simulink model "GT_trim"  (R2024a)
settings: Solver=ode4  StartTime=0.0  StopTime=t(end)  FixedStep=1/1600  RelTol=1e-3
undefined symbols (not defined in the file): wind_x, wind_y, wind_z
libraries: Sensors x4, GT x1
settings Model: Creator=igmso  LastModifiedBy=igmso
settings DataIOCC: ExternalInput=[t,u]  InitialState=getstatestruct(op_trim3)  LoadExternalInput=on  SaveFormat=StructureWithTime

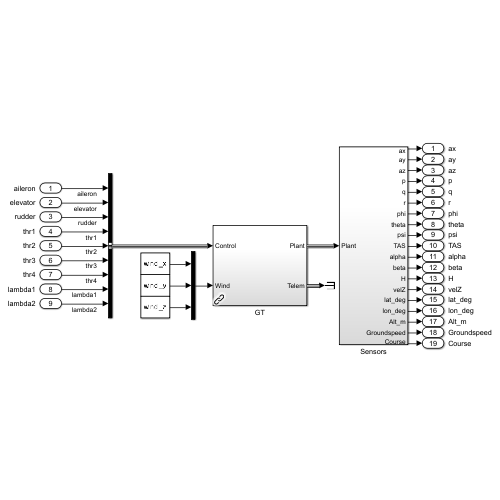
[thumbnail: Simulink's stored preview of the top-level diagram]
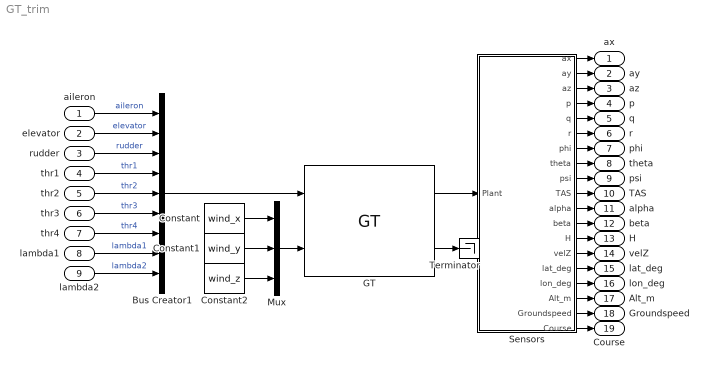
== system GT_trim ==
  aileron : Inport
  elevator : Inport  Port=2
  rudder : Inport  Port=3
  thr1 : Inport  Port=4
  thr2 : Inport  Port=5
  thr3 : Inport  Port=6
  thr4 : Inport  Port=7
  lambda1 : Inport  Port=8
  lambda2 : Inport  Port=9
  Bus Creator1 : BusCreator  Inputs=9
  Constant : Constant  Value=wind_x
  Constant1 : Constant  Value=wind_y
  Constant2 : Constant  Value=wind_z
  GT : GT/GT  SystemSampleTime=-1  VariantActivationTime=update diagram  AllowFlexibleInterface=on  Latency=0  AutoFrameSizeCalculation=off
  Mux : Mux  Inputs=3
  Sensors : Subsystem
  Terminator : Terminator
  ax : Outport
  ay : Outport  Port=2
  az : Outport  Port=3
  p : Outport  Port=4
  q : Outport  Port=5
  r : Outport  Port=6
  phi : Outport  Port=7
  theta : Outport  Port=8
  psi : Outport  Port=9
  TAS : Outport  Port=10
  alpha : Outport  Port=11
  beta : Outport  Port=12
  H : Outport  Port=13
  velZ : Outport  Port=14
  lat_deg : Outport  Port=15
  lon_deg : Outport  Port=16
  Alt_m : Outport  Port=17
  Groundspeed : Outport  Port=18
  Course : Outport  Port=19
  wires:
  Bus Creator1/1 -> GT/1
  lambda2/1 -> Bus Creator1/9  "lambda2"
  lambda1/1 -> Bus Creator1/8  "lambda1"
  thr2/1 -> Bus Creator1/5  "thr2"
  thr3/1 -> Bus Creator1/6  "thr3"
  rudder/1 -> Bus Creator1/3  "rudder"
  thr1/1 -> Bus Creator1/4  "thr1"
  elevator/1 -> Bus Creator1/2  "elevator"
  aileron/1 -> Bus Creator1/1  "aileron"
  thr4/1 -> Bus Creator1/7  "thr4"
  Mux/1 -> GT/2
  Constant/1 -> Mux/1
  Constant1/1 -> Mux/2
  Constant2/1 -> Mux/3
  GT/2 -> Terminator/1
  Sensors/8(theta) -> theta/1
  Sensors/13(H) -> H/1
  Sensors/7(phi) -> phi/1
  Sensors/3(az) -> az/1
  GT/1 -> Sensors/1(Plant)
  Sensors/9(psi) -> psi/1
  Sensors/1(ax) -> ax/1
  Sensors/2(ay) -> ay/1
  Sensors/11(alpha) -> alpha/1
  Sensors/6(r) -> r/1
  Sensors/5(q) -> q/1
  Sensors/4(p) -> p/1
  Sensors/12(beta) -> beta/1
  Sensors/10(TAS) -> TAS/1
  Sensors/16(lon_deg) -> lon_deg/1
  Sensors/14(velZ) -> velZ/1
  Sensors/15(lat_deg) -> lat_deg/1
  Sensors/17(Alt_m) -> Alt_m/1
  Sensors/18(Groundspeed) -> Groundspeed/1
  Sensors/19(Course) -> Course/1

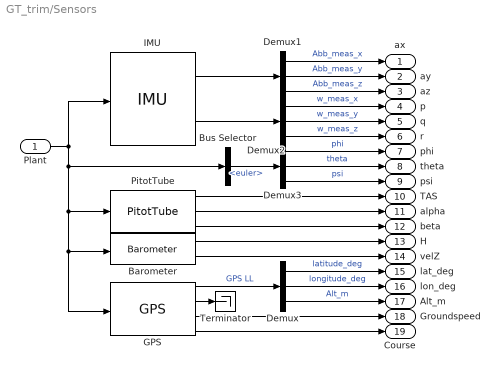
== system GT_trim/Sensors ==
  Plant : Inport
  Barometer : Sensors/Barometer  SystemSampleTime=1/400  VariantActivationTime=update diagram  AllowFlexibleInterface=on  Latency=0  AutoFrameSizeCalculation=off
  Bus Selector : BusSelector  OutputSignals=euler
  Demux{,1..3} (4 alike) : Demux  Outputs=3
  GPS : Sensors/GPS  SystemSampleTime=1/400  VariantActivationTime=update diagram  AllowFlexibleInterface=on  Latency=0  AutoFrameSizeCalculation=off
  IMU : Sensors/IMU  SystemSampleTime=-1  VariantActivationTime=update diagram  AllowFlexibleInterface=on  Latency=0  AutoFrameSizeCalculation=off
  PitotTube : Sensors/PitotTube  SystemSampleTime=1/400  VariantActivationTime=update diagram  AllowFlexibleInterface=on  Latency=0  AutoFrameSizeCalculation=off
  Terminator : Terminator
  ax : Outport
  ay : Outport  Port=2
  az : Outport  Port=3
  p : Outport  Port=4
  q : Outport  Port=5
  r : Outport  Port=6
  phi : Outport  Port=7
  theta : Outport  Port=8
  psi : Outport  Port=9
  TAS : Outport  Port=10
  alpha : Outport  Port=11
  beta : Outport  Port=12
  H : Outport  Port=13
  velZ : Outport  Port=14
  lat_deg : Outport  Port=15
  lon_deg : Outport  Port=16
  Alt_m : Outport  Port=17
  Groundspeed : Outport  Port=18
  Course : Outport  Port=19
  wires:
  Barometer/1 -> H/1
  GPS/2 -> Terminator/1
  GPS/3 -> Groundspeed/1
  GPS/4 -> Course/1
  Plant/1 -> GPS/1, Barometer/1, PitotTube/1, Bus Selector/1, IMU/1
  Demux/1 -> lat_deg/1  "latitude_deg"
  Demux/2 -> lon_deg/1  "longitude_deg"
  Demux/3 -> Alt_m/1  "Alt_m"
  PitotTube/1 -> TAS/1
  PitotTube/2 -> alpha/1
  PitotTube/3 -> beta/1
  Demux1/3 -> az/1  "Abb_meas_z"
  Demux1/2 -> ay/1  "Abb_meas_y"
  Demux1/1 -> ax/1  "Abb_meas_x"
  IMU/1 -> Demux1/1
  IMU/2 -> Demux2/1
  Demux2/1 -> p/1  "w_meas_x"
  Demux2/2 -> q/1  "w_meas_y"
  Demux2/3 -> r/1  "w_meas_z"
  Barometer/2 -> velZ/1
  GPS/1 -> Demux/1  "GPS LL"
  Bus Selector/1 -> Demux3/1  "<euler>"
  Demux3/1 -> phi/1  "phi"
  Demux3/2 -> theta/1  "theta"
  Demux3/3 -> psi/1  "psi"
